simulink model "stop_fsm"  (R2022a)
settings: Solver=FixedStepDiscrete  StartTime=0.0  StopTime=10.0  FixedStep=0.1  RelTol=1e-3  EnableMultiTasking=on
settings Model: Creator=steve  LastModifiedBy=steve
settings SolverCC: AlgebraicLoopSolver=TrustRegion  AutoInsertRateTranBlk=on
settings DataIOCC: LimitDataPoints=on
settings OptimizationCC: LifeSpan=inf
settings DebuggingCC: UnconnectedInputMsg=warning  UnconnectedOutputMsg=warning  UnconnectedLineMsg=warning  AllowSymbolicDim=off  SFUnexpectedBacktrackingDiag=warning  SFNoUnconditionalDefaultTransitionDiag=warning  SFExecutionAtInitializationDiag=none  ArithmeticOperatorsInVariantConditions=warning
settings SFSimCC: SimUseLocalCustomCode=off  CustomCodeUndefinedFunction=UseInterfaceOnly
settings RTWCC: RTWUseLocalCustomCode=off  DLArmComputeVersion=19.05
settings CodeAppCC: StateflowObjectComments=on
settings GRTTargetCC: TargetLangStandard=C89/C90 (ANSI)
settings ConfigComp: CovMetricSettings=dw  CovSaveCumulativeToWorkspaceVar=on  CovSaveSingleToWorkspaceVar=on  CovExternalEMLEnable=off  CovSFcnEnable=off

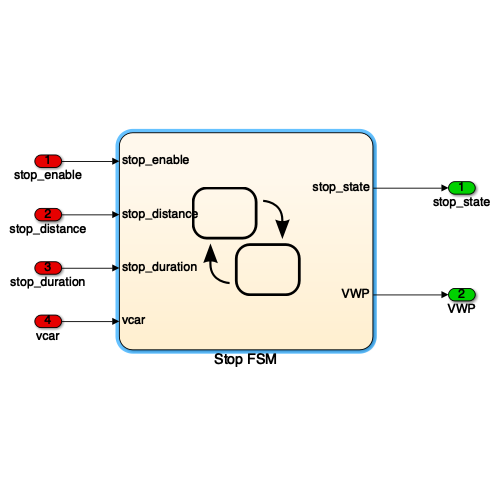
[thumbnail: Simulink's stored preview of the top-level diagram]
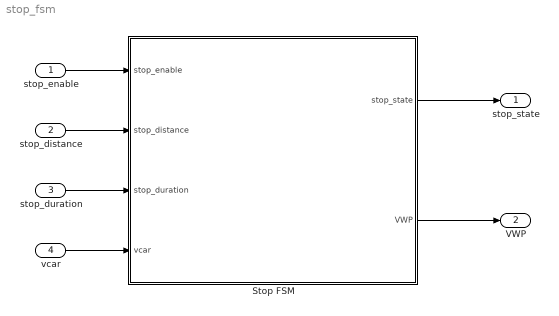
== system stop_fsm ==
  stop_enable : Inport
  stop_distance : Inport  Port=2
  stop_duration : Inport  Port=3
  vcar : Inport  Port=4
  Stop FSM : Stateflow chart  TreatAsAtomicUnit=on
  stop_state : Outport
  VWP : Outport  Port=2
  wires:
  stop_enable/1 -> Stop FSM/1(stop_enable)
  stop_distance/1 -> Stop FSM/2(stop_distance)
  stop_duration/1 -> Stop FSM/3(stop_duration)
  vcar/1 -> Stop FSM/4(vcar)
  Stop FSM/1(stop_state) -> stop_state/1
  Stop FSM/2(VWP) -> VWP/1

== stateflow chart stop_fsm/Stop FSM ==
  state wait_for_stop_enable
    en:  stop_state = 0;
  state wait_for_zero_velocity
    en:  stop_state = 1;
  state wait_for_stop_duration
    en:  stop_state = 2;
    du:  tnow = get_current_time();
  (default) -> wait_for_stop_enable
  wait_for_stop_enable -> wait_for_stop_enable [order 2]
  wait_for_stop_duration -> wait_for_stop_enable [order 1] : [tnow >= tstop || stop_enable == false]
  wait_for_zero_velocity -> wait_for_stop_enable [order 1] : [stop_enable == false]
  wait_for_stop_enable -> wait_for_zero_velocity [order 1] : [stop_enable == true]
      | {VWP = update_VWP(stop_distance,VWP)}
  wait_for_zero_velocity -> wait_for_zero_velocity [order 3]
  wait_for_zero_velocity -> wait_for_stop_duration [order 2] : [vcar == 0]
      | {tstop = stop_duration + get_current_time();}
  wait_for_stop_duration -> wait_for_stop_duration [order 2]
  data: stop_enable input; stop_distance input; stop_duration input; stop_state output; VWP output; vcar input; tstop local; tnow local
